simulink model "Robot_gravity"  (R2024b)
settings: Solver=VariableStepAuto  StartTime=0.0  StopTime=10.0  RelTol=1e-3
values from neighbouring files (symbols this model uses):
  robot = loadrobot('kukaIiwa14', 'DataFormat', 'column')    [Corioli.m]    (also in Mass_Matrix.m; ext_force.m; min_max_torques.m = loadrobot('kukaIiwa14', 'DataFormat', 'column', 'Gravity', [)
undefined symbols (not defined in the file or in its folder): conf
libraries: robotmaniplib x1, simulink_extras x1
settings Model: Creator=mloukili  LastModifiedBy=mloukili

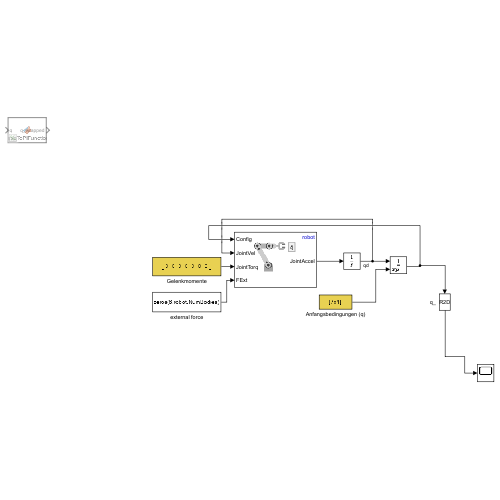
[thumbnail: Simulink's stored preview of the top-level diagram]
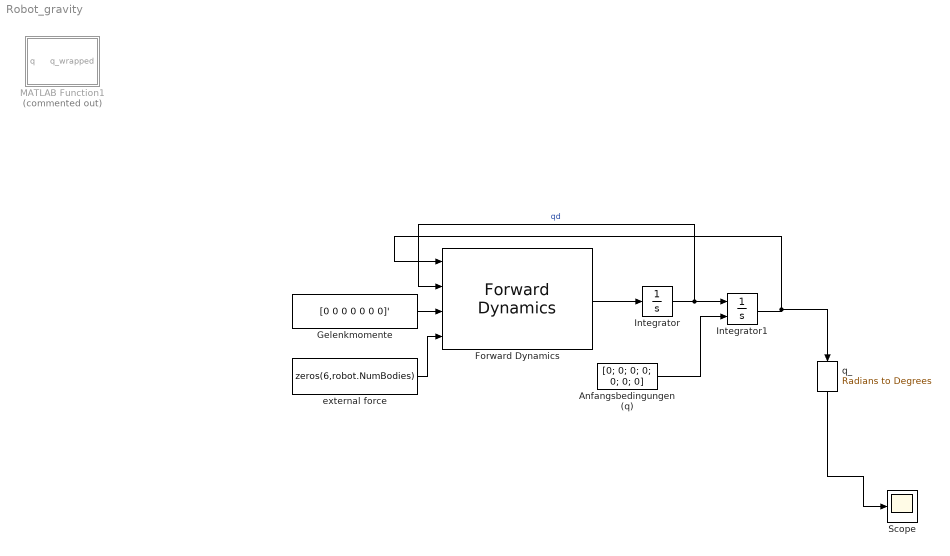
== system Robot_gravity ==
  Anfangsbedingungen (q) : Constant  Value=[0; 0; 0; 0; 0; 0; 0]
  Forward Dynamics : robotmaniplib/Forward Dynamics  RigidBodyTree=robot  SimulateUsing=Interpreted execution
  Gelenkmomente : Constant  Value=[0 0 0 0 0 0 0]'
  Integrator : Integrator
  Integrator1 : Integrator  InitialConditionSource=external  InitialCondition=conf.qs
  MATLAB Function1 : MATLAB Function  Commented=on  TreatAsAtomicUnit=on
  Scope : Scope
  external force : Constant  Value=zeros(6,robot.NumBodies)
  q_ : simulink_extras/Transformations/Radians to Degrees
  wires:
  Gelenkmomente/1 -> Forward Dynamics/3
  external force/1 -> Forward Dynamics/4
  Forward Dynamics/1 -> Integrator/1
  Integrator/1 -> Forward Dynamics/2, Integrator1/1  "qd"
  Anfangsbedingungen (q)/1 -> Integrator1/2
  q_/1 -> Scope/1
  Integrator1/1 -> q_/1, Forward Dynamics/1

== matlab function Robot_gravity/MATLAB Function1 ==
  data: q input; q_wrapped output
function q_wrapped = wrapToPiFunction(q)
    q_wrapped = wrapToPi(q);
end
